simulink model "SingleAgent_Simulink"  (R2024b)
settings: Solver=VariableStepAuto  StartTime=0.0  StopTime=10.0  RelTol=1e-3
settings Model: Creator=panat  LastModifiedBy=panat

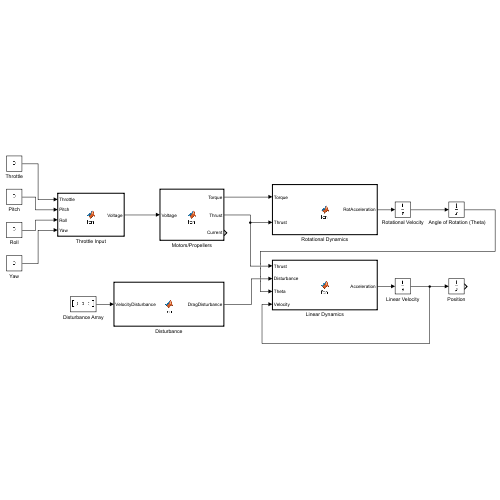
[thumbnail: Simulink's stored preview of the top-level diagram]
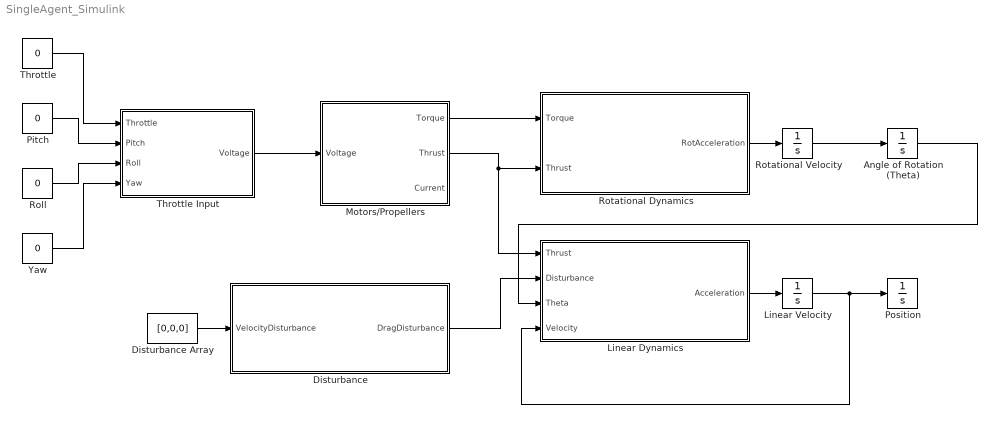
== system SingleAgent_Simulink ==
  " Angle of Rotation (Theta)" : Integrator
  Disturbance : MATLAB Function  TreatAsAtomicUnit=on
  Disturbance Array : Constant  Value=[0,0,0]
  Linear Dynamics : MATLAB Function  TreatAsAtomicUnit=on
  Linear Velocity : Integrator
  Motors/Propellers : MATLAB Function  TreatAsAtomicUnit=on
  Pitch : Constant  Value=0
  Position : Integrator
  Roll : Constant  Value=0
  Rotational Dynamics : MATLAB Function  TreatAsAtomicUnit=on
  Rotational Velocity : Integrator
  Throttle : Constant  Value=0
  Throttle Input : MATLAB Function  TreatAsAtomicUnit=on
  Yaw : Constant  Value=0
  wires:
  Motors/Propellers/1(Torque) -> Rotational Dynamics/1(Torque)
  Motors/Propellers/2(Thrust) -> Linear Dynamics/1(Thrust), Rotational Dynamics/2(Thrust)
  Rotational Dynamics/1(RotAcceleration) -> Rotational Velocity/1
  Rotational Velocity/1 -> " Angle of Rotation (Theta)"/1
  " Angle of Rotation (Theta)"/1 -> Linear Dynamics/3(Theta)
  Linear Dynamics/1(Acceleration) -> Linear Velocity/1
  Linear Velocity/1 -> Linear Dynamics/4(Velocity), Position/1
  Disturbance/1(DragDisturbance) -> Linear Dynamics/2(Disturbance)
  Disturbance Array/1 -> Disturbance/1(VelocityDisturbance)
  Throttle Input/1(Voltage) -> Motors/Propellers/1(Voltage)
  Throttle/1 -> Throttle Input/1(Throttle)
  Pitch/1 -> Throttle Input/2(Pitch)
  Roll/1 -> Throttle Input/3(Roll)
  Yaw/1 -> Throttle Input/4(Yaw)

== matlab function SingleAgent_Simulink/Rotational Dynamics ==
  data: Torque input; RotAcceleration output; Thrust input
function RotAcceleration = fcn(Torque, Thrust)
Moment=[0 0 0];
RotAcceleration=[0 0 0];
Inertia=[0.003,0.003,0.007];
Moment(1)=(Thrust(3)+Thrust(4))*0.237/2-(Thrust(1)+Thrust(2))*0.237/2;
Moment(2)=(Thrust(3)+Thrust(2))*0.237/2-(Thrust(1)+Thrust(4))*0.237/2;
Moment(3)=Torque(4)-Torque(1)+Torque(2)-Torque(3);
for i=1:3
    RotAcceleration(i)=Moment(i)/Inertia(i);
end

== matlab function SingleAgent_Simulink/Motors//Propellers ==
  data: Voltage input; Torque output; Thrust output; Current output
function [Torque, Thrust, Current] = fcn(Voltage)
RPM=[0 0 0 0];
Torque=[0 0 0 0];
Current=[0 0 0 0];
Thrust=[0 0 0 0];
for i=1:4
    RPM(i)=-2.6931*Voltage(i)^3+1400*Voltage(i);
    Ct=2*10^-15*RPM(i)^3-4*10^-11*RPM(i)^2+3*10^-7*RPM(i)+0.1013;
    Thrust(i)=Ct*1.225*(RPM(i)/60)^2*0.2^4;
    Torque(i)=4*10^-14*RPM(i)^3+8*10^-12*RPM(i)^2+3*10-6*RPM(i);
    Current(i)=1400*Torque(i);
end

== matlab function SingleAgent_Simulink/Linear Dynamics ==
  data: Thrust input; Acceleration output; Disturbance input; Theta input; Velocity input
function Acceleration = fcn(Thrust, Disturbance, Theta, Velocity)
m=0.743;
g=9.81;
A=[0.197 0.197 0.0512];
rho=1.225;
Cd=1;

Acceleration=[0 0 0];
Force=[0 0 0];
Fprop=[0 0 0];

Fprop(1)=sin(Theta(2))*cos(Theta(1))*(Thrust(1)+Thrust(2)+Thrust(3)+Thrust(4));
Fprop(2)=sin(Theta(1))*cos(Theta(2))*(Thrust(1)+Thrust(2)+Thrust(3)+Thrust(4));
Fprop(3)=cos(Theta(1))*cos(Theta(2))*(Thrust(1)+Thrust(2)+Thrust(3)+Thrust(4));

ThetaXY=atan2(Fprop(1),Fprop(2));
XY2D=sqrt(Fprop(1)^2+Fprop(2)^2);
if Fprop(3)>=0
    Fprop(1)=XY2D*sin(Theta(3)+ThetaXY);
    Fprop(2)=XY2D*cos(Theta(3)+ThetaXY);
else
    Fprop(1)=XY2D*sin(-Theta(3)+ThetaXY);
    Fprop(2)=XY2D*cos(-Theta(3)+ThetaXY);
end

if Velocity(1)<0
    Force(1)=Fprop(1)-Disturbance(1)+0.5*rho*Velocity(1)^2*A(1)*Cd;
else
    Force(1)=Fprop(1)-Disturbance(1)-0.5*rho*Velocity(1)^2*A(1)*Cd;
end

if Velocity(2)<0
    Force(2)=Fprop(2)-Disturbance(2)+0.5*rho*Velocity(2)^2*A(2)*Cd;
else
    Force(2)=Fprop(2)-Disturbance(2)-0.5*rho*Velocity(2)^2*A(2)*Cd;
end

if Velocity(3)<0
    Force(3)=Fprop(3)-Disturbance(3)+0.5*rho*Velocity(3)^2*A(3)*Cd-m*g;
else
    Force(3)=Fprop(3)-Disturbance(3)-0.5*rho*Velocity(3)^2*A(3)*Cd-m*g;
end

for i=1:3
    Acceleration(i)=Force(i)/m;
end

== matlab function SingleAgent_Simulink/Disturbance ==
  data: VelocityDisturbance input; DragDisturbance output
function DragDisturbance = fcn(VelocityDisturbance)
A=[0.0197 0.0197 0.0197*2*1.3]; %projected area
DragDisturbance=[0 0 0];
rho=1.225 %air density at sea level
Cd=1; %drag coefficient 

for i=1:3
    if VelocityDisturbance(i)<0
        DragDisturbance(i)=-0.5*rho*VelocityDisturbance(i)^2*A(i)*Cd;
    else
        DragDisturbance(i)=0.5*rho*VelocityDisturbance(i)^2*A(i)*Cd;
    end
end

== matlab function SingleAgent_Simulink/Throttle Input ==
  data: Throttle input; Voltage output; Pitch input; Roll input; Yaw input
function Voltage = fcn(Throttle, Pitch, Roll, Yaw)
Correct=0; %correction variable
Vbatt=11.4; %battery voltage
%throttling correction
if (Pitch/2+Roll/2+Yaw/2)>(100-Throttle)%maximum throttling as percentage
    Correct=((Pitch/2+Roll/2+Yaw/2)-(100-Throttle));
end
if (Pitch/2+Roll/2+Yaw/2)>(Throttle)%minimum throttling as percentage
    if Correct<((Pitch/2+Roll/2+Yaw/2)-(Throttle))
        Correct=((Pitch/2+Roll/2+Yaw/2)-(Throttle));
    end
end

%pitch roll yaw correction
if Correct~=0
Pitch=Pitch-Correct/3*2;
Roll=Roll-Correct/3*2;
Yaw=Yaw-Correct/3*2;
end 

%motor voltage regulator
Voltage=[(Throttle-Pitch/2-Roll/2-Yaw/2)*Vbatt/100
    (Throttle-Pitch/2+Roll/2+Yaw/2)*Vbatt/100
    (Throttle+Pitch/2+Roll/2-Yaw/2)*Vbatt/100
    (Throttle+Pitch/2-Roll/2-Yaw/2)*Vbatt/100];
